simulink model "pv_frictionmodel"  (R2018b)
settings: configuration reference "Physics" (kept outside this file)
model workspace (MAT data in the model file):
  veh_param = Simulink.Parameter
  veh_param.Value.cLiftF = 0
  veh_param.Value.cLiftR = 0
  veh_param.Value.CoGx_m = 0
  veh_param.Value.CoGy_m = 0
  veh_param.Value.CoGz_m = 0
  veh_param.Value.cDrag = 0
  veh_param.Value.Aref_m2 = 0
  veh_param.Value.Gearratio = 0
  veh_param.Value.Wheelbase_m = 0
  veh_param.Value.PacLatF = [0 0 0 0 0]
  veh_param.Value.PacLongF = [0 0 0 0 0]
  veh_param.Value.PacLatR = [0 0 0 0 0]
  veh_param.Value.PacLongR = [0 0 0 0 0]
  veh_param.Value.cRollFriction_Npmps = 0
  veh_param.Value.MaxRollFriction_N = 0
  veh_param.Value.T_YawRate_s = 0
  veh_param.Value.T_LatVel_s = 0
  veh_param.Value.TrackWidthF_m = 0
  veh_param.Value.TrackWidthR_m = 0
  veh_param.Value.TireRadiusF_m = 0
  veh_param.Value.TireRadiusR_m = 0
  veh_param.Value.VehicleInertia_kgm2 = 0
  veh_param.Value.WheelInertiaF_kgm2 = 0
  veh_param.Value.WheelInertiaR_kgm2 = 0
  veh_param.Value.VehicleMass_kg = 0
  veh_param.Value.switchModelBlend_mps = 0
  veh_param.Value.PTLimitLowVel_N = 0
  veh_param.Value.switchModelVel_mps = 0
  veh_param.Value.T_Tire_s = 0
  veh_param.DataType = 'struct'
  veh_param.Dimensions = [1 1]
  x0_positionstates = Simulink.Parameter
  x0_positionstates.Value = [0 0 0]
  x0_positionstates.DataType = 'auto'
  x0_positionstates.Dimensions = [1 3]
undefined symbols (not defined in the file): VEH__VehicleData__l_WheelbaseF_m, VEH__VehicleData__l_WheelbaseTotal_m, VEH__VehicleData__w_TrackF_m, VEH__VehicleData__w_TrackR_m
settings Model: DataDictionary=frictionmodel.sldd  OrderedModelArguments=off  Creator=wischnewski  LastModifiedBy=staer

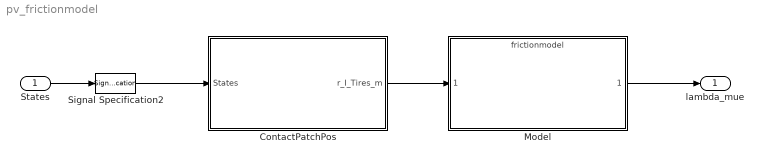
== system pv_frictionmodel ==
  States : Inport
  ContactPatchPos : MATLAB Function  TreatAsAtomicUnit=on
  Model : ModelReference  ModelNameDialog=frictionmodel.slx  SimulationMode=Normal  ModelReferenceVersion=1.355
  Signal Specification2 : SignalSpecification  Dimensions=[1,3]
  lambda_mue : Outport
  wires:
  States/1 -> Signal Specification2/1
  ContactPatchPos/1(r_I_Tires_m) -> Model/1
  Model/1 -> lambda_mue/1
  Signal Specification2/1 -> ContactPatchPos/1(States)

== matlab function pv_frictionmodel/ContactPatchPos ==
  data: States input; r_I_Tires_m output size=[3 4]; VEH__VehicleData__l_WheelbaseF_m parameter; VEH__VehicleData__l_WheelbaseTotal_m parameter; VEH__VehicleData__w_TrackF_m parameter; VEH__VehicleData__w_TrackR_m parameter
function r_I_Tires_m  = fcn(States, ...
    VEH__VehicleData__l_WheelbaseF_m, VEH__VehicleData__l_WheelbaseTotal_m, ...
    VEH__VehicleData__w_TrackF_m, VEH__VehicleData__w_TrackR_m)

[r_I_Tires_m] = ContactPatchPos(States, ...
    VEH__VehicleData__l_WheelbaseF_m, VEH__VehicleData__l_WheelbaseTotal_m, ...
    VEH__VehicleData__w_TrackF_m, VEH__VehicleData__w_TrackR_m);
